simulink library "SimOneModule"  (Simulink 9.1)
settings: Solver=VariableStepAuto  StartTime=0.0  StopTime=10.0  RelTol=1e-3
settings Model: Creator=xuliang  LastModifiedBy=panpan

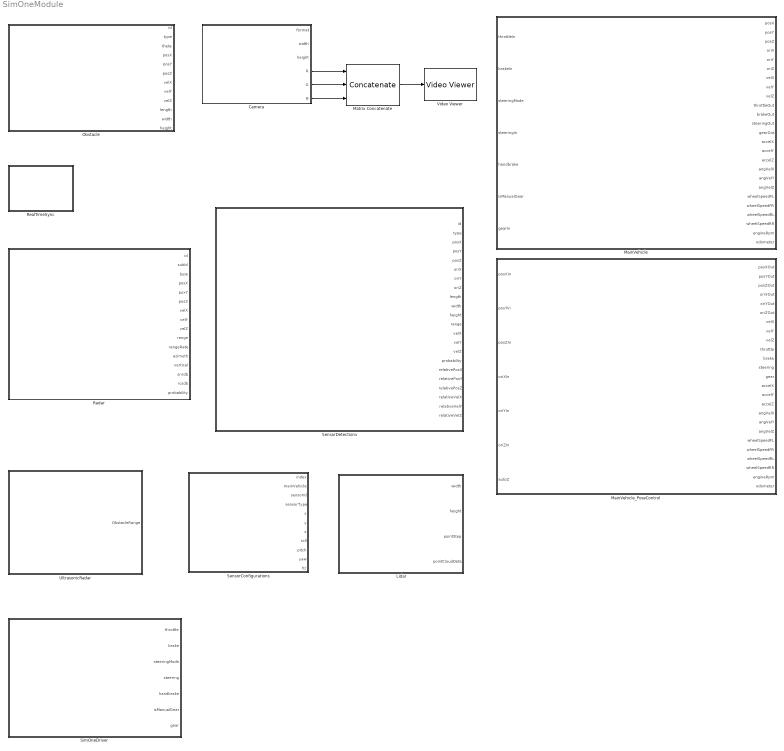
== system SimOneModule ==
  Camera : Subsystem  mask(SimOne Source Block: Camera){IP="127.0.0.1", Port=5566, CameraId=1, HorizontalResolution=1920, VerticalResolution=1080}
      mask help:
      | Get Image Data
      |
      | @Parameter
      | CameraId: Camera index in SimOne
      |
      | HorizontalResolution: Image resolution width, configure of sensor camera on web UI
      |
      | VerticalResolution: Image resolution height, configure of sensor camera on web UI
      |
      | @Output
      | [format, width, height, R, G, B]
  Lidar : Subsystem  mask(SimOne Source Block: Lidar){IP="127.0.0.1", Port=7788, LidarId=1, MaxPointCloudDataSize=3686400}
      mask prompts: MaxPointCloudDataSize "PointCloudDataSize"
      mask help:
      | Get PointCloud Data
      |
      | @Parameter
      | LidarId: Lidar index in SimOne
      |
      | PointCloudDataSize: Max pointcloud data size
      |
      | @Output
      | [width, height, pointStep, pointCloudData]: PointCloud data(ouput)
  MainVehicle : Subsystem  mask(SimOne Source Block: MainVehicle){}
      mask help:
      | Get main vehicle GPS
      |
      | @Input
      | Control: vehicle control data(input)
      |
      | @Output
      | GPS data(output)
  MainVehicle_PoseControl : Subsystem  mask(SimOne Source Block: MainVehicle_PoseControl){}
      mask help:
      | Set main vehicle pose
      |
      | @Input
      | PoseControl: Pose to set(input)
      |
      | @Output
      | GPS Data(output)
  Matrix Concatenate : Concatenate  NumInputs=3  Mode=Multidimensional array  ConcatenateDimension=3
  Obstacle : Subsystem  mask(SimOne Source Block: Obstacle){MaxObstacleNum=100, ObstacleId=1}
      mask prompts: MaxObstacleNum "ObstacleNum"
      mask help:
      | Get Ground Truth Data of Objects(Obstacles) from simulation scene
      |
      | @Parameter
      | ObstacleNum: Max detected obstacle number
      |
      | ObstacleId: Obstacle index, starts from 1
      |
      | @Output
      | Obstacle data(output)
  Radar : Subsystem  mask(SimOne Source Block: Radar){RadarId=1, MaxRadarDetectNum=200, RadarDetectionsId=1}
      mask prompts: MaxRadarDetectNum "RadarDetectNum"
      mask help:
      | Get millimeter wave radar detections
      |
      | @Parameter
      | RadarId: Radar index in SimOne
      |
      | RadarDetectNum: Max Radar detected obstacle number
      |
      | RadarDetectionsId: Obstacle index, starts from 1
      |
      | @Output
      | Radar detections(output)
  RealTimeSync : Subsystem  mask(SimOne Source Block: RealTimeSync){}
      mask help: Perform model's real-time simulation without any additional components
  "SensorConfigurations " : Subsystem  mask(SimOne Source Block: SensorConfigurations){MaxSensorNum=10, SensorConfigId=1}
      mask prompts: MaxSensorNum "SensorNum"
      mask help:
      | Get Sensor's position information
      |
      | @Parameter
      | SensorNum: Max sensor number
      |
      | SensorConfigId: Sensor index, starts from 1
      |
      | @Output
      | SensorConfig: SensorConfigurations data (output)
  SensorDetections : Subsystem  mask(SimOne Source Block: SensorDetections){SensorId=1, MaxSensorDetectNum=100, SensorDetectionsId=1}
      mask prompts: MaxSensorDetectNum "SensorDetectNum"
      mask help:
      | Get Ground Truth objects for current sensor, support camera, lidar and perfect perception sensors
      |
      | @Parameter
      | SensorId: Sensor index in SimOne
      |
      | SensorDetectNum: Max sensor detected obstacle number
      |
      | SensorDetectionsId: Obstacle index, starts from 1
      |
      | @Output
      | SensorDetectData: SimOne_Data_SensorDetections data(output)
  SimOneDriver : Subsystem  mask(SimOne Source Block: SimOneDriver){}
      mask help:
      | Get vehicle control data from SimOneDriver
      |
      | @Output
      | Control: vehicle control data(input)
  UltrasonicRadar : Subsystem  mask(SimOne Source Block: UltrasonicRadar){UltrasonicRadarId=1, MaxUltrasonicDetectNum=100, UltrasonicDetectionsId=1}
      mask prompts: MaxUltrasonicDetectNum "UltrasonicDetectNum"
      mask help:
      | Get UltrasonicRadar imformations
      |
      | @Parameter
      | UltrasonicRadarId: UltrasonicRadar index in SimOne
      |
      | UltrasonicDetectNum: Max Ultrasonic detected obstacle number
      |
      | UltrasonicDetectionsId: Obstacle index, starts from 1
      |
      | @Output
      | Ultrasonic data in SimOne_Data_UltrasonicRadar format(output)
  Video Viewer : VideoViewer  FigPos=[2041 741 418 304]
  wires:
  Camera/5(G) -> Matrix Concatenate/2
  Camera/4(R) -> Matrix Concatenate/1
  Camera/6(B) -> Matrix Concatenate/3
  Matrix Concatenate/1 -> Video Viewer/1

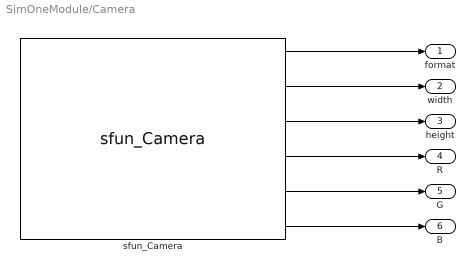
== system SimOneModule/Camera ==
  sfun_Camera : S-Function  FunctionName=sfun_Camera  Parameters=IP Port CameraId HorizontalResolution VerticalResolution  SFunctionDeploymentMode=off  EnableBusSupport=off
  format : Outport
  "width " : Outport  Port=2
  "height " : Outport  Port=3
  R : Outport  Port=4
  G : Outport  Port=5
  B : Outport  Port=6
  wires:
  sfun_Camera/1 -> format/1
  sfun_Camera/2 -> "width "/1
  sfun_Camera/3 -> "height "/1
  sfun_Camera/4 -> R/1
  sfun_Camera/5 -> G/1
  sfun_Camera/6 -> B/1

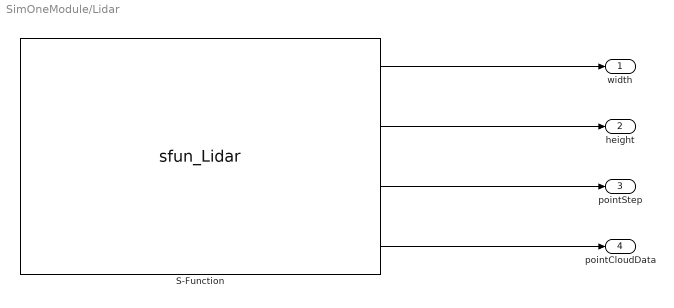
== system SimOneModule/Lidar ==
  S-Function : S-Function  FunctionName=sfun_Lidar  Parameters=IP Port LidarId MaxPointCloudDataSize  SFunctionDeploymentMode=off  EnableBusSupport=off
  width : Outport
  height : Outport  Port=2
  pointStep : Outport  Port=3
  pointCloudData : Outport  Port=4
  wires:
  S-Function/1 -> width/1
  S-Function/2 -> height/1
  S-Function/3 -> pointStep/1
  S-Function/4 -> pointCloudData/1

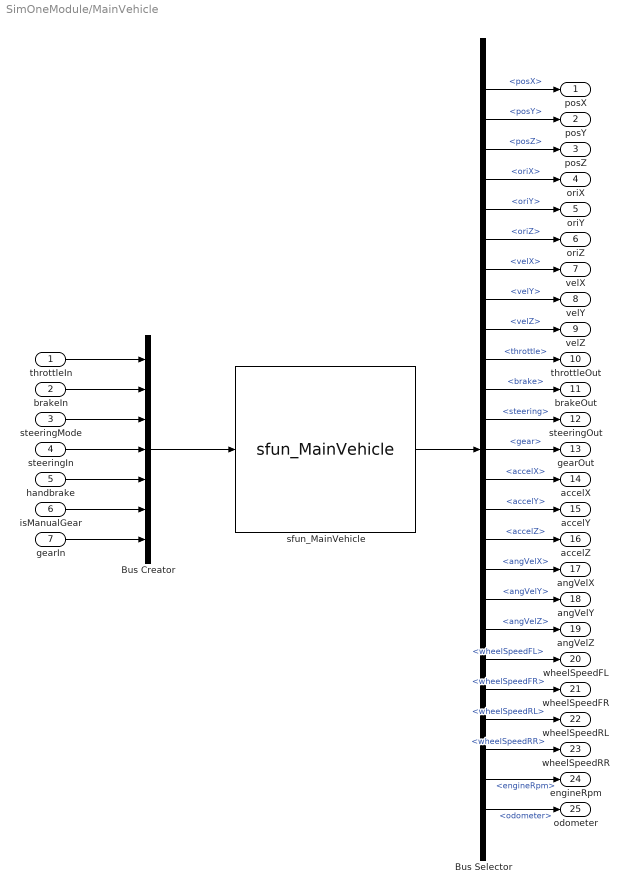
== system SimOneModule/MainVehicle ==
  throttleIn : Inport  OutDataTypeStr=single
  brakeIn : Inport  Port=2  OutDataTypeStr=single
  steeringMode : Inport  Port=3  OutDataTypeStr=int32
  steeringIn : Inport  Port=4  OutDataTypeStr=single
  "handbrake " : Inport  Port=5  OutDataTypeStr=boolean
  isManualGear : Inport  Port=6  OutDataTypeStr=boolean
  gearIn : Inport  Port=7  OutDataTypeStr=int32
  Bus Creator : BusCreator  Inputs=7  OutDataTypeStr=Bus: SimOne_Data_Control_Bus
      settings: InheritFromInputs=off
  Bus Selector : BusSelector  OutputSignals=posX,posY,posZ,oriX,oriY,oriZ,velX,velY,velZ,throttle,brake,steering,gear,accelX,accelY,accelZ,angVelX,angVelY,angVelZ,wheelSpeedFL,wheelSpeedFR,wheelSpeedRL,wheelSpeedRR,engineRpm,odometer
  sfun_MainVehicle : S-Function  FunctionName=sfun_MainVehicle  SFunctionDeploymentMode=off  EnableBusSupport=off
  posX : Outport
  posY : Outport  Port=2
  posZ : Outport  Port=3
  oriX : Outport  Port=4
  oriY : Outport  Port=5
  oriZ : Outport  Port=6
  velX : Outport  Port=7
  velY : Outport  Port=8
  velZ : Outport  Port=9
  throttleOut : Outport  Port=10
  brakeOut : Outport  Port=11
  steeringOut : Outport  Port=12
  gearOut : Outport  Port=13
  accelX : Outport  Port=14
  accelY : Outport  Port=15
  accelZ : Outport  Port=16
  angVelX : Outport  Port=17
  angVelY : Outport  Port=18
  angVelZ : Outport  Port=19
  wheelSpeedFL : Outport  Port=20
  wheelSpeedFR : Outport  Port=21
  wheelSpeedRL : Outport  Port=22
  wheelSpeedRR : Outport  Port=23
  engineRpm : Outport  Port=24
  odometer : Outport  Port=25
  wires:
  Bus Selector/1 -> posX/1  "<posX>"
  Bus Selector/2 -> posY/1  "<posY>"
  Bus Selector/3 -> posZ/1  "<posZ>"
  Bus Selector/4 -> oriX/1  "<oriX>"
  Bus Selector/5 -> oriY/1  "<oriY>"
  Bus Selector/6 -> oriZ/1  "<oriZ>"
  Bus Selector/7 -> velX/1  "<velX>"
  Bus Selector/8 -> velY/1  "<velY>"
  Bus Selector/9 -> velZ/1  "<velZ>"
  Bus Selector/10 -> throttleOut/1  "<throttle>"
  Bus Selector/11 -> brakeOut/1  "<brake>"
  Bus Selector/12 -> steeringOut/1  "<steering>"
  Bus Selector/13 -> gearOut/1  "<gear>"
  Bus Selector/14 -> accelX/1  "<accelX>"
  Bus Selector/15 -> accelY/1  "<accelY>"
  Bus Selector/16 -> accelZ/1  "<accelZ>"
  Bus Selector/17 -> angVelX/1  "<angVelX>"
  Bus Selector/18 -> angVelY/1  "<angVelY>"
  Bus Selector/19 -> angVelZ/1  "<angVelZ>"
  Bus Selector/20 -> wheelSpeedFL/1  "<wheelSpeedFL>"
  Bus Selector/21 -> wheelSpeedFR/1  "<wheelSpeedFR>"
  Bus Selector/22 -> wheelSpeedRL/1  "<wheelSpeedRL>"
  Bus Selector/23 -> wheelSpeedRR/1  "<wheelSpeedRR>"
  throttleIn/1 -> Bus Creator/1
  brakeIn/1 -> Bus Creator/2
  steeringMode/1 -> Bus Creator/3
  "handbrake "/1 -> Bus Creator/5
  isManualGear/1 -> Bus Creator/6
  gearIn/1 -> Bus Creator/7
  sfun_MainVehicle/1 -> Bus Selector/1
  Bus Creator/1 -> sfun_MainVehicle/1
  Bus Selector/24 -> engineRpm/1  "<engineRpm>"
  Bus Selector/25 -> odometer/1  "<odometer>"
  steeringIn/1 -> Bus Creator/4

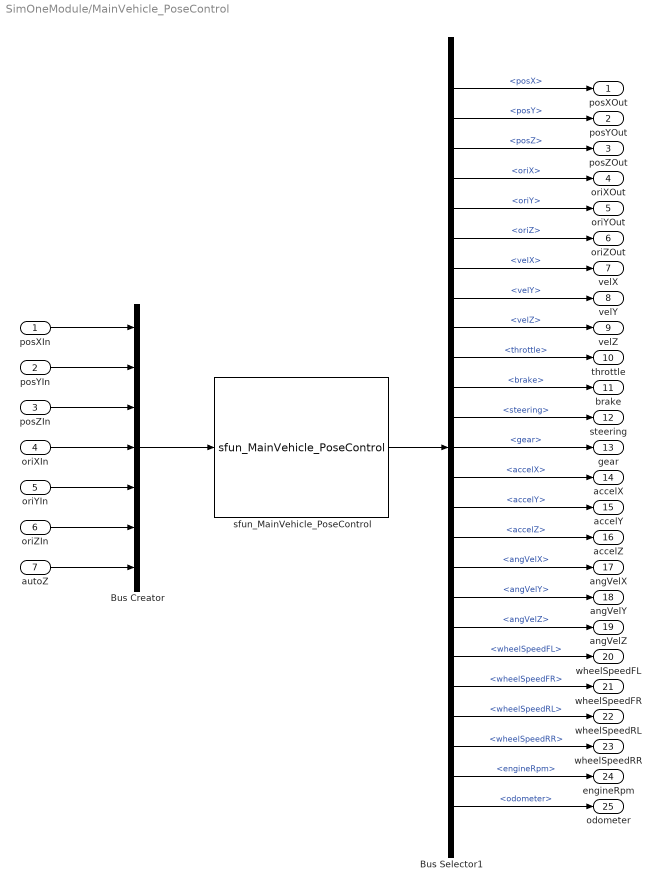
== system SimOneModule/MainVehicle_PoseControl ==
  posXIn : Inport
  posYIn : Inport  Port=2
  posZIn : Inport  Port=3
  oriXIn : Inport  Port=4
  oriYIn : Inport  Port=5
  oriZIn : Inport  Port=6
  autoZ : Inport  Port=7
  Bus Creator : BusCreator  Inputs=7  OutDataTypeStr=Bus: SimOne_Data_Pose_Control_Bus
      settings: InheritFromInputs=off
  Bus Selector1 : BusSelector  OutputSignals=posX,posY,posZ,oriX,oriY,oriZ,velX,velY,velZ,throttle,brake,steering,gear,accelX,accelY,accelZ,angVelX,angVelY,angVelZ,wheelSpeedFL,wheelSpeedFR,wheelSpeedRL,wheelSpeedRR,engineRpm,odometer
  sfun_MainVehicle_PoseControl : S-Function  FunctionName=sfun_MainVehicle_PoseControl  SFunctionDeploymentMode=off  EnableBusSupport=off
  posXOut : Outport
  posYOut : Outport  Port=2
  posZOut : Outport  Port=3
  oriXOut : Outport  Port=4
  oriYOut : Outport  Port=5
  oriZOut : Outport  Port=6
  velX : Outport  Port=7
  velY : Outport  Port=8
  velZ : Outport  Port=9
  throttle : Outport  Port=10
  brake : Outport  Port=11
  steering : Outport  Port=12
  gear : Outport  Port=13
  accelX : Outport  Port=14
  accelY : Outport  Port=15
  accelZ : Outport  Port=16
  angVelX : Outport  Port=17
  angVelY : Outport  Port=18
  angVelZ : Outport  Port=19
  wheelSpeedFL : Outport  Port=20
  wheelSpeedFR : Outport  Port=21
  wheelSpeedRL : Outport  Port=22
  wheelSpeedRR : Outport  Port=23
  engineRpm : Outport  Port=24
  odometer : Outport  Port=25
  wires:
  Bus Selector1/20 -> wheelSpeedFL/1  "<wheelSpeedFL>"
  Bus Selector1/22 -> wheelSpeedRL/1  "<wheelSpeedRL>"
  Bus Selector1/23 -> wheelSpeedRR/1  "<wheelSpeedRR>"
  Bus Selector1/2 -> posYOut/1  "<posY>"
  Bus Selector1/1 -> posXOut/1  "<posX>"
  Bus Selector1/7 -> velX/1  "<velX>"
  Bus Selector1/5 -> oriYOut/1  "<oriY>"
  Bus Selector1/8 -> velY/1  "<velY>"
  Bus Selector1/6 -> oriZOut/1  "<oriZ>"
  Bus Selector1/13 -> gear/1  "<gear>"
  Bus Selector1/12 -> steering/1  "<steering>"
  Bus Selector1/17 -> angVelX/1  "<angVelX>"
  Bus Selector1/10 -> throttle/1  "<throttle>"
  Bus Selector1/3 -> posZOut/1  "<posZ>"
  Bus Selector1/18 -> angVelY/1  "<angVelY>"
  Bus Selector1/11 -> brake/1  "<brake>"
  Bus Selector1/21 -> wheelSpeedFR/1  "<wheelSpeedFR>"
  Bus Selector1/16 -> accelZ/1  "<accelZ>"
  Bus Selector1/15 -> accelY/1  "<accelY>"
  Bus Selector1/4 -> oriXOut/1  "<oriX>"
  sfun_MainVehicle_PoseControl/1 -> Bus Selector1/1
  Bus Selector1/19 -> angVelZ/1  "<angVelZ>"
  Bus Selector1/14 -> accelX/1  "<accelX>"
  Bus Selector1/9 -> velZ/1  "<velZ>"
  posXIn/1 -> Bus Creator/1
  autoZ/1 -> Bus Creator/7
  oriZIn/1 -> Bus Creator/6
  oriYIn/1 -> Bus Creator/5
  oriXIn/1 -> Bus Creator/4
  posYIn/1 -> Bus Creator/2
  posZIn/1 -> Bus Creator/3
  Bus Creator/1 -> sfun_MainVehicle_PoseControl/1
  Bus Selector1/24 -> engineRpm/1  "<engineRpm>"
  Bus Selector1/25 -> odometer/1  "<odometer>"

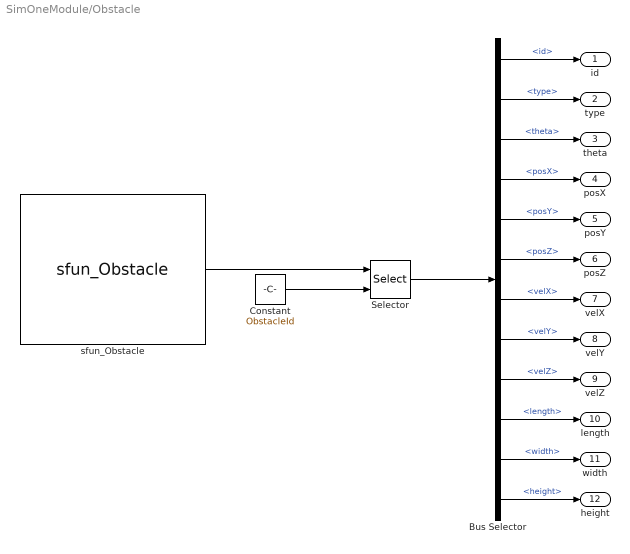
== system SimOneModule/Obstacle ==
  Bus Selector : BusSelector  OutputSignals=id,type,theta,posX,posY,posZ,velX,velY,velZ,length,width,height
  Constant : Constant  Value=ObstacleId
  Selector : Selector  InputPortWidth=MaxObstacleNum  IndexOptions=Index vector (port)  Indices=[1 3]  OutputSizes=1
  sfun_Obstacle : S-Function  FunctionName=sfun_Obstacle  Parameters=MaxObstacleNum  SFunctionDeploymentMode=off  EnableBusSupport=off
  id : Outport
  type : Outport  Port=2
  theta : Outport  Port=3
  posX : Outport  Port=4
  posY : Outport  Port=5
  posZ : Outport  Port=6
  velX : Outport  Port=7
  velY : Outport  Port=8
  velZ : Outport  Port=9
  length : Outport  Port=10
  width : Outport  Port=11
  height : Outport  Port=12
  wires:
  sfun_Obstacle/1 -> Selector/1
  Selector/1 -> Bus Selector/1
  Constant/1 -> Selector/2
  Bus Selector/1 -> id/1  "<id>"
  Bus Selector/12 -> height/1  "<height>"
  Bus Selector/11 -> width/1  "<width>"
  Bus Selector/10 -> length/1  "<length>"
  Bus Selector/9 -> velZ/1  "<velZ>"
  Bus Selector/8 -> velY/1  "<velY>"
  Bus Selector/7 -> velX/1  "<velX>"
  Bus Selector/6 -> posZ/1  "<posZ>"
  Bus Selector/5 -> posY/1  "<posY>"
  Bus Selector/4 -> posX/1  "<posX>"
  Bus Selector/3 -> theta/1  "<theta>"
  Bus Selector/2 -> type/1  "<type>"

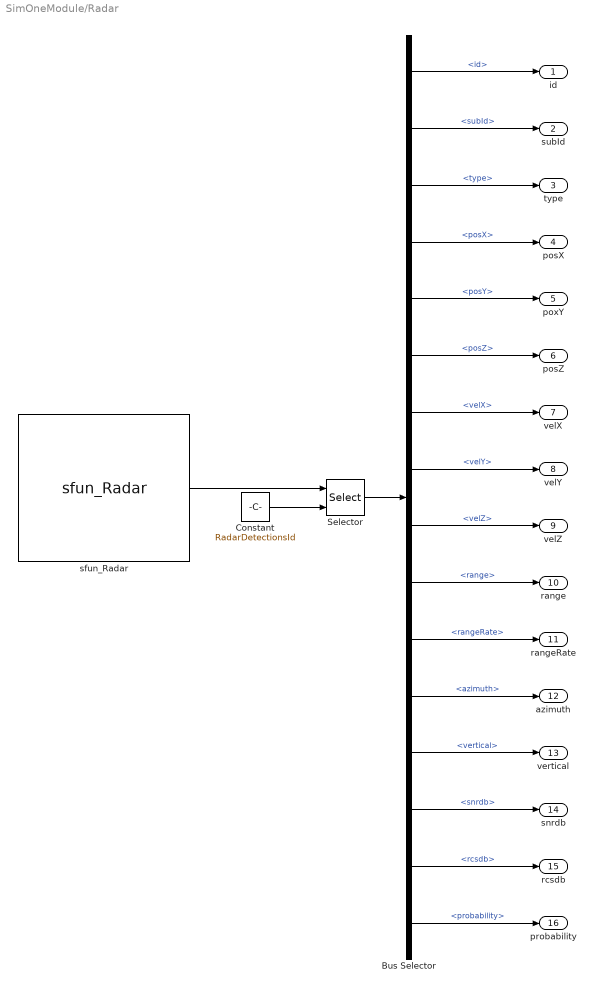
== system SimOneModule/Radar ==
  Bus Selector : BusSelector  OutputSignals=id,subId,type,posX,posY,posZ,velX,velY,velZ,range,rangeRate,azimuth,vertical,snrdb,rcsdb,probability
  Constant : Constant  Value=RadarDetectionsId
  Selector : Selector  InputPortWidth=MaxRadarDetectNum  IndexOptions=Index vector (port)  Indices=[1 3]  OutputSizes=1
  "sfun_Radar " : S-Function  FunctionName=sfun_Radar  Parameters=RadarId MaxRadarDetectNum  SFunctionDeploymentMode=off  EnableBusSupport=off
  id : Outport
  subId : Outport  Port=2
  type : Outport  Port=3
  posX : Outport  Port=4
  poxY : Outport  Port=5
  posZ : Outport  Port=6
  velX : Outport  Port=7
  velY : Outport  Port=8
  velZ : Outport  Port=9
  range : Outport  Port=10
  rangeRate : Outport  Port=11
  azimuth : Outport  Port=12
  vertical : Outport  Port=13
  snrdb : Outport  Port=14
  rcsdb : Outport  Port=15
  probability : Outport  Port=16
  wires:
  "sfun_Radar "/1 -> Selector/1
  Constant/1 -> Selector/2
  Selector/1 -> Bus Selector/1
  Bus Selector/1 -> id/1  "<id>"
  Bus Selector/2 -> subId/1  "<subId>"
  Bus Selector/3 -> type/1  "<type>"
  Bus Selector/4 -> posX/1  "<posX>"
  Bus Selector/5 -> poxY/1  "<posY>"
  Bus Selector/6 -> posZ/1  "<posZ>"
  Bus Selector/7 -> velX/1  "<velX>"
  Bus Selector/8 -> velY/1  "<velY>"
  Bus Selector/9 -> velZ/1  "<velZ>"
  Bus Selector/11 -> rangeRate/1  "<rangeRate>"
  Bus Selector/12 -> azimuth/1  "<azimuth>"
  Bus Selector/13 -> vertical/1  "<vertical>"
  Bus Selector/10 -> range/1  "<range>"
  Bus Selector/14 -> snrdb/1  "<snrdb>"
  Bus Selector/15 -> rcsdb/1  "<rcsdb>"
  Bus Selector/16 -> probability/1  "<probability>"

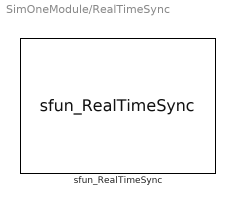
== system SimOneModule/RealTimeSync ==
  sfun_RealTimeSync : S-Function  FunctionName=sfun_RealTimeSync  SFunctionDeploymentMode=off  EnableBusSupport=off

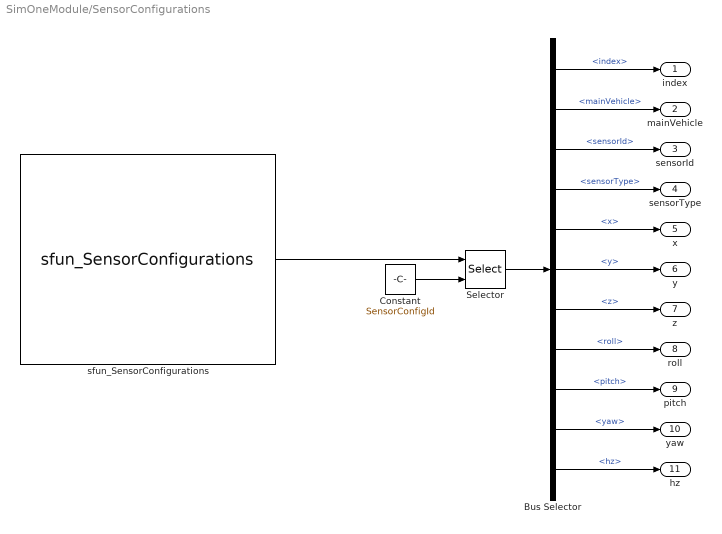
== system SimOneModule/SensorConfigurations  ==
  Bus Selector : BusSelector  OutputSignals=index,mainVehicle,sensorId,sensorType,x,y,z,roll,pitch,yaw,hz
  Constant : Constant  Value=SensorConfigId
  Selector : Selector  InputPortWidth=10  IndexOptions=Index vector (port)  Indices=[1 3]  OutputSizes=1
  sfun_SensorConfigurations : S-Function  FunctionName=sfun_SensorConfigurations  Parameters=MaxSensorNum  SFunctionDeploymentMode=off  EnableBusSupport=off
  index : Outport
  "mainVehicle " : Outport  Port=2
  sensorId : Outport  Port=3
  sensorType : Outport  Port=4
  x : Outport  Port=5
  y : Outport  Port=6
  z : Outport  Port=7
  roll : Outport  Port=8
  pitch : Outport  Port=9
  yaw : Outport  Port=10
  hz : Outport  Port=11
  wires:
  sfun_SensorConfigurations/1 -> Selector/1
  Constant/1 -> Selector/2
  Selector/1 -> Bus Selector/1
  Bus Selector/2 -> "mainVehicle "/1  "<mainVehicle>"
  Bus Selector/3 -> sensorId/1  "<sensorId>"
  Bus Selector/11 -> hz/1  "<hz>"
  Bus Selector/10 -> yaw/1  "<yaw>"
  Bus Selector/9 -> pitch/1  "<pitch>"
  Bus Selector/8 -> roll/1  "<roll>"
  Bus Selector/7 -> z/1  "<z>"
  Bus Selector/6 -> y/1  "<y>"
  Bus Selector/5 -> x/1  "<x>"
  Bus Selector/1 -> index/1  "<index>"
  Bus Selector/4 -> sensorType/1  "<sensorType>"

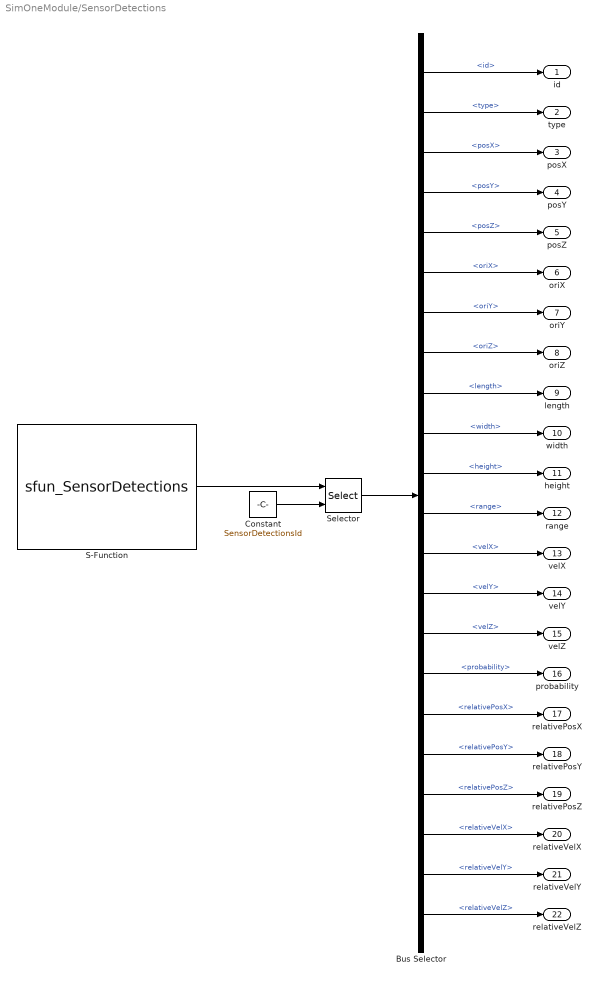
== system SimOneModule/SensorDetections ==
  Bus Selector : BusSelector  OutputSignals=id,type,posX,posY,posZ,oriX,oriY,oriZ,length,width,height,range,velX,velY,velZ,probability,relativePosX,relativePosY,relativePosZ,relativeVelX,relativeVelY,relativeVelZ
  Constant : Constant  Value=SensorDetectionsId
  S-Function : S-Function  FunctionName=sfun_SensorDetections  Parameters=SensorId MaxSensorDetectNum  SFunctionDeploymentMode=off  EnableBusSupport=off
  Selector : Selector  InputPortWidth=MaxSensorDetectNum  IndexOptions=Index vector (port)  Indices=[1 3]  OutputSizes=1
  id : Outport
  type : Outport  Port=2
  posX : Outport  Port=3
  posY : Outport  Port=4
  posZ : Outport  Port=5
  oriX : Outport  Port=6
  oriY : Outport  Port=7
  oriZ : Outport  Port=8
  length : Outport  Port=9
  width : Outport  Port=10
  height : Outport  Port=11
  range : Outport  Port=12
  velX : Outport  Port=13
  velY : Outport  Port=14
  velZ : Outport  Port=15
  probability : Outport  Port=16
  relativePosX : Outport  Port=17
  relativePosY : Outport  Port=18
  relativePosZ : Outport  Port=19
  relativeVelX : Outport  Port=20
  relativeVelY : Outport  Port=21
  relativeVelZ : Outport  Port=22
  wires:
  S-Function/1 -> Selector/1
  Constant/1 -> Selector/2
  Selector/1 -> Bus Selector/1
  Bus Selector/1 -> id/1  "<id>"
  Bus Selector/2 -> type/1  "<type>"
  Bus Selector/3 -> posX/1  "<posX>"
  Bus Selector/4 -> posY/1  "<posY>"
  Bus Selector/5 -> posZ/1  "<posZ>"
  Bus Selector/6 -> oriX/1  "<oriX>"
  Bus Selector/7 -> oriY/1  "<oriY>"
  Bus Selector/8 -> oriZ/1  "<oriZ>"
  Bus Selector/9 -> length/1  "<length>"
  Bus Selector/10 -> width/1  "<width>"
  Bus Selector/11 -> height/1  "<height>"
  Bus Selector/12 -> range/1  "<range>"
  Bus Selector/13 -> velX/1  "<velX>"
  Bus Selector/14 -> velY/1  "<velY>"
  Bus Selector/15 -> velZ/1  "<velZ>"
  Bus Selector/16 -> probability/1  "<probability>"
  Bus Selector/17 -> relativePosX/1  "<relativePosX>"
  Bus Selector/18 -> relativePosY/1  "<relativePosY>"
  Bus Selector/19 -> relativePosZ/1  "<relativePosZ>"
  Bus Selector/20 -> relativeVelX/1  "<relativeVelX>"
  Bus Selector/21 -> relativeVelY/1  "<relativeVelY>"
  Bus Selector/22 -> relativeVelZ/1  "<relativeVelZ>"

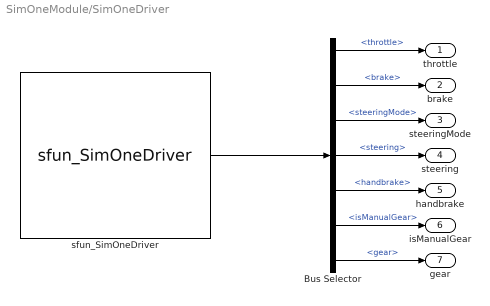
== system SimOneModule/SimOneDriver ==
  Bus Selector : BusSelector  OutputSignals=throttle,brake,steeringMode,steering,handbrake,isManualGear,gear
  sfun_SimOneDriver : S-Function  FunctionName=sfun_SimOneDriver  SFunctionDeploymentMode=off  EnableBusSupport=off
  throttle : Outport
  brake : Outport  Port=2
  steeringMode : Outport  Port=3
  steering : Outport  Port=4
  handbrake : Outport  Port=5
  isManualGear : Outport  Port=6
  gear : Outport  Port=7
  wires:
  sfun_SimOneDriver/1 -> Bus Selector/1
  Bus Selector/1 -> throttle/1  "<throttle>"
  Bus Selector/2 -> brake/1  "<brake>"
  Bus Selector/4 -> steering/1  "<steering>"
  Bus Selector/5 -> handbrake/1  "<handbrake>"
  Bus Selector/6 -> isManualGear/1  "<isManualGear>"
  Bus Selector/7 -> gear/1  "<gear>"
  Bus Selector/3 -> steeringMode/1  "<steeringMode>"

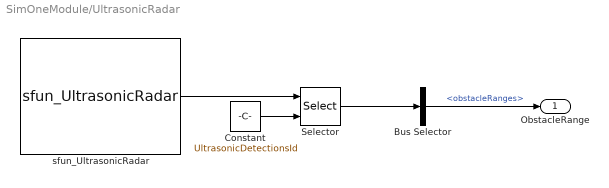
== system SimOneModule/UltrasonicRadar ==
  Bus Selector : BusSelector  OutputSignals=obstacleRanges
  Constant : Constant  Value=UltrasonicDetectionsId
  Selector : Selector  InputPortWidth=MaxUltrasonicDetectNum  IndexOptions=Index vector (port)  Indices=[1 3]  OutputSizes=1
  "sfun_UltrasonicRadar " : S-Function  FunctionName=sfun_UltrasonicRadar  Parameters=UltrasonicRadarId MaxUltrasonicDetectNum  SFunctionDeploymentMode=off  EnableBusSupport=off
  ObstacleRange : Outport
  wires:
  "sfun_UltrasonicRadar "/1 -> Selector/1
  Constant/1 -> Selector/2
  Selector/1 -> Bus Selector/1
  Bus Selector/1 -> ObstacleRange/1  "<obstacleRanges>"
